simulink model "four_CIFF_EM_sim"  (R2020a)
settings: Solver=VariableStepAuto  StartTime=0.0  StopTime=0.2  MaxStep=1.55424749113179e-06  RelTol=0.0001
values from neighbouring files (symbols this model uses):
  a = [1 -1]    [CIC_Filter.m]    (also in Cascade_CIC_Filter.m; four_CIFF_EM.m = 0.9)
  Amax = 8    [four_CIFF_EM.m]
  Amp1 = 10*5.13e-6    (= 5.13e-05)    [four_CIFF_EM.m]
  finrad = Fin*2*pi    (= 188.495559215)    [four_CIFF_EM.m]
  g1 = 0.4    [four_CIFF_EM.m]
  g2 = 0.2    [four_CIFF_EM.m]
  g3 = 4    [four_CIFF_EM.m]
  g4 = 0.9    [four_CIFF_EM.m]
  GAIN = 50    [four_CIFF_EM.m]
  Kcv = 4e12    (= 4000000000000)    [four_CIFF_EM.m]
  Kvf = 1.323e-4    (= 0.0001323)    [four_CIFF_EM.m]
  n = length(w)    [CIC_Filter.m]    (also in Cascade_CIC_Filter.m; Half_Band_Filter.m = 18; four_CIFF_EM.m = 0.08)
  Ts = 1/Fs    (= 1.953125e-06)    [four_CIFF_EM.m]
  Vref = 1    [four_CIFF_EM.m]
  ws = sqrt(k/m)    [four_CIFF_EM.m]
libraries: SDtoolbox x1
(part 1 of 3)
settings Model: Creator=Chuqby  LastModifiedBy=Chuqby
settings DataIOCC: ReturnWorkspaceOutputs=off

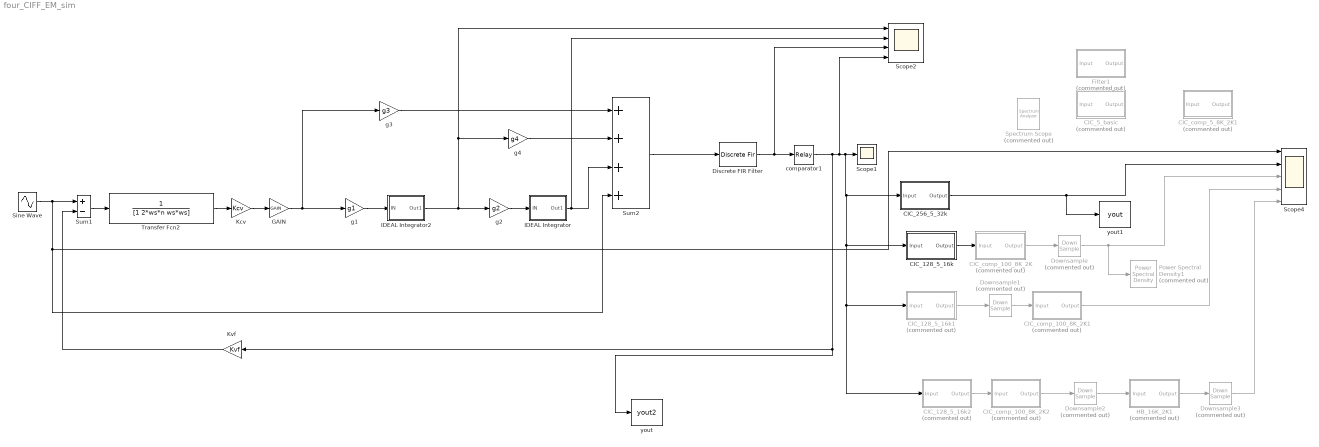
== system four_CIFF_EM_sim ==
  CIC_128_5_16k : Subsystem  Tag=FilterWizardSubSystem
      settings: ErrorFcn=dspFilterRealizedInBasicElemsAlgLoopErrFcnCallback
  CIC_128_5_16k1 : Subsystem  Tag=FilterWizardSubSystem  Commented=on
      settings: ErrorFcn=dspFilterRealizedInBasicElemsAlgLoopErrFcnCallback
  CIC_128_5_16k2 : Subsystem  Tag=FilterWizardSubSystem  Commented=on
      settings: ErrorFcn=dspFilterRealizedInBasicElemsAlgLoopErrFcnCallback
  CIC_256_5_32k : Subsystem  Tag=FilterWizardSubSystem
      settings: ErrorFcn=dspFilterRealizedInBasicElemsAlgLoopErrFcnCallback
  CIC_5_basic : Subsystem  Tag=FilterWizardSubSystem  Commented=on
      settings: ErrorFcn=dspFilterRealizedInBasicElemsAlgLoopErrFcnCallback
  CIC_comp_100_8K_2K : Subsystem  Tag=FilterWizardSubSystem  Commented=on
      settings: ErrorFcn=dspFilterRealizedInBasicElemsAlgLoopErrFcnCallback
  CIC_comp_100_8K_2K1 : Subsystem  Tag=FilterWizardSubSystem  Commented=on
      settings: ErrorFcn=dspFilterRealizedInBasicElemsAlgLoopErrFcnCallback
  CIC_comp_100_8K_2K2 : Subsystem  Tag=FilterWizardSubSystem  Commented=on
      settings: ErrorFcn=dspFilterRealizedInBasicElemsAlgLoopErrFcnCallback
  CIC_comp_5_8K_2K1 : Subsystem  Tag=FilterWizardSubSystem  Commented=on
      settings: ErrorFcn=dspFilterRealizedInBasicElemsAlgLoopErrFcnCallback
  Discrete FIR Filter : DiscreteFir  Coefficients=[1 -a]  SampleTime=Ts
  Downsample{,1..3} (4 alike) : DownSample  Commented=on  RateOptions=Allow multirate processing
  Filter1 : Subsystem  Tag=FilterWizardSubSystem  Commented=on
      settings: ErrorFcn=dspFilterRealizedInBasicElemsAlgLoopErrFcnCallback
  GAIN : Gain  Gain=GAIN
  HB_16K_2K1 : Subsystem  Tag=FilterWizardSubSystem  Commented=on
      settings: ErrorFcn=dspFilterRealizedInBasicElemsAlgLoopErrFcnCallback
  IDEAL Integrator : Subsystem  mask(Integrator){Amax=Amax, Ts=Ts}
      mask prompts: Amax "Saturation"; Ts "Sample Time:"
      mask help:
      | Real discrete integrator with delay.
      | Models op-amp saturation and slew rate.
      mask Help:
      | Parameters:
      | Ts:       Sample time
      | G:         Finite op-amp gain (ideal op-amp G=1)
      | Amax:  Saturation value
      | sr:       slew rate in V/s
      mask Display: dpoly([0 1], [1 -1], 'z-')
  IDEAL Integrator2 : Subsystem  mask(Integrator){Amax=Amax, Ts=Ts}
      mask prompts: Amax "Saturation"; Ts "Sample Time:"
      mask help:
      | Real discrete integrator with delay.
      | Models op-amp saturation and slew rate.
      mask Help:
      | Parameters:
      | Ts:       Sample time
      | G:         Finite op-amp gain (ideal op-amp G=1)
      | Amax:  Saturation value
      | sr:       slew rate in V/s
      mask Display: dpoly([0 1], [1 -1], 'z-')
  Kcv : Gain  Gain=Kcv
  Kvf : Gain  Gain=Kvf
  Power Spectral Density1 : SDtoolbox/Power Spectral Density  Commented=on  SN=1  Fs=8000  fBL=1  fBH=2000  Fin=30  N=65535  Ntransient=Ntransient  VW=off  savename=savemat  Scale_type=logarithmic
  Scope1 : Scope
  Scope2 : Scope  NumInputPorts=4
  Scope4 : Scope  NumInputPorts=5
  Sine Wave : Sin  Amplitude=Amp1  Frequency=finrad  SampleTime=0
  Spectrum Scope : SpectrumAnalyzer  Commented=on
  Sum1 : Sum  Inputs=+-
  Sum2 : Sum  Inputs=++++
  Transfer Fcn2 : TransferFcn  Denominator=[1 2*ws*n ws*ws]
  comparator1 : Relay  OnOutputValue=Vref  OffOutputValue=-Vref  ZeroCross=off
  g1 : Gain  Gain=g1
  g2 : Gain  Gain=g2
  g3 : Gain  Gain=g3
  g4 : Gain  Gain=g4
  yout : ToWorkspace  VariableName=yout2  SampleTime=-1
      settings: Save2DSignal=2-D array (concatenate along first dimension)
  yout1 : ToWorkspace  VariableName=yout  SampleTime=-1
      settings: Save2DSignal=2-D array (concatenate along first dimension)
  wires:
  IDEAL Integrator2/1(Out1) -> Scope2/1, g4/1, g2/1
  g3/1 -> Sum2/1
  g4/1 -> Sum2/2
  Sum1/1 -> Transfer Fcn2/1
  Discrete FIR Filter/1 -> Scope2/3, comparator1/1
  g1/1 -> IDEAL Integrator2/1(IN)
  g2/1 -> IDEAL Integrator/1(IN)
  Sum2/1 -> Discrete FIR Filter/1
  Transfer Fcn2/1 -> Kcv/1
  IDEAL Integrator/1(Out1) -> Sum2/3, Scope2/2
  Sine Wave/1 -> Scope4/1, Sum2/4, Sum1/1
  Kcv/1 -> GAIN/1
  comparator1/1 -> Scope2/4, CIC_256_5_32k/1(Input), CIC_128_5_16k2/1(Input), CIC_128_5_16k1/1(Input), CIC_128_5_16k/1(Input), Scope1/1, yout/1, Kvf/1
  GAIN/1 -> g1/1, g3/1
  Kvf/1 -> Sum1/2
  CIC_256_5_32k/1(Output) -> yout1/1, Scope4/2
  CIC_128_5_16k/1(Output) -> CIC_comp_100_8K_2K/1(Input)
  CIC_comp_100_8K_2K/1(Output) -> Downsample/1
  Downsample/1 -> Power Spectral Density1/1, Scope4/3
  CIC_128_5_16k1/1(Output) -> Downsample1/1
  Downsample1/1 -> CIC_comp_100_8K_2K1/1(Input)
  CIC_comp_100_8K_2K1/1(Output) -> Scope4/4
  CIC_comp_100_8K_2K2/1(Output) -> Downsample2/1
  CIC_128_5_16k2/1(Output) -> CIC_comp_100_8K_2K2/1(Input)
  Downsample2/1 -> HB_16K_2K1/1(Input)
  Downsample3/1 -> Scope4/5
  HB_16K_2K1/1(Output) -> Downsample3/1

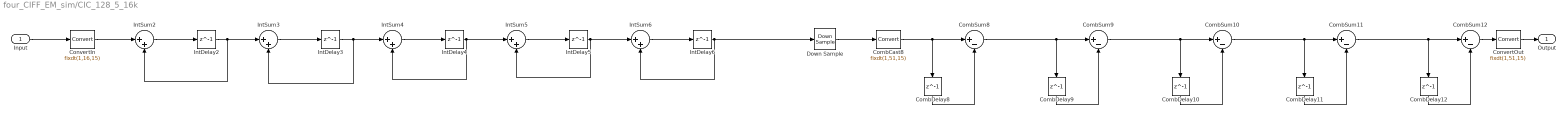
== system four_CIFF_EM_sim/CIC_128_5_16k ==
  Input : Inport
  CombCast8 : DataTypeConversion  OutDataTypeStr=fixdt(1,51,15)
  CombDelay{8..12} (5 alike) : Delay  DelayLength=1  InitialCondition=0
  CombSum{8..12} (5 alike) : Sum  Inputs=|+-  AccumDataTypeStr=fixdt(1,51,15)  OutDataTypeStr=fixdt(1,51,15)
  ConvertIn : DataTypeConversion  OutDataTypeStr=fixdt(1,16,15)  RndMeth=Nearest  SaturateOnIntegerOverflow=on
  ConvertOut : DataTypeConversion  OutDataTypeStr=fixdt(1,51,15)
  Down Sample : DownSample  N=128  RateOptions=Allow multirate processing
  IntDelay{2..6} (5 alike) : Delay  DelayLength=1  InitialCondition=0
  IntSum{2..6} (5 alike) : Sum  Inputs=|++  AccumDataTypeStr=fixdt(1,51,15)  OutDataTypeStr=fixdt(1,51,15)
  Output : Outport
  wires:
  Input/1 -> ConvertIn/1
  ConvertIn/1 -> IntSum2/1
  IntSum2/1 -> IntDelay2/1
  IntDelay2/1 -> IntSum2/2, IntSum3/1
  IntSum3/1 -> IntDelay3/1
  IntDelay3/1 -> IntSum3/2, IntSum4/1
  IntSum4/1 -> IntDelay4/1
  IntDelay4/1 -> IntSum4/2, IntSum5/1
  IntSum5/1 -> IntDelay5/1
  IntDelay5/1 -> IntSum5/2, IntSum6/1
  IntSum6/1 -> IntDelay6/1
  IntDelay6/1 -> IntSum6/2, Down Sample/1
  Down Sample/1 -> CombCast8/1
  CombSum8/1 -> CombSum9/1, CombDelay9/1
  CombDelay8/1 -> CombSum8/2
  CombCast8/1 -> CombSum8/1, CombDelay8/1
  CombSum9/1 -> CombSum10/1, CombDelay10/1
  CombDelay9/1 -> CombSum9/2
  CombSum10/1 -> CombSum11/1, CombDelay11/1
  CombDelay10/1 -> CombSum10/2
  CombSum11/1 -> CombSum12/1, CombDelay12/1
  CombDelay11/1 -> CombSum11/2
  CombSum12/1 -> ConvertOut/1
  CombDelay12/1 -> CombSum12/2
  ConvertOut/1 -> Output/1

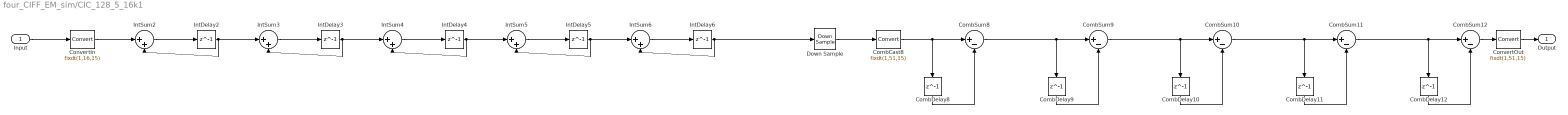
== system four_CIFF_EM_sim/CIC_128_5_16k1 ==
  Input : Inport
  CombCast8 : DataTypeConversion  OutDataTypeStr=fixdt(1,51,15)
  CombDelay{8..12} (5 alike) : Delay  DelayLength=1  InitialCondition=0
  CombSum{8..12} (5 alike) : Sum  Inputs=|+-  AccumDataTypeStr=fixdt(1,51,15)  OutDataTypeStr=fixdt(1,51,15)
  ConvertIn : DataTypeConversion  OutDataTypeStr=fixdt(1,16,15)  RndMeth=Nearest  SaturateOnIntegerOverflow=on
  ConvertOut : DataTypeConversion  OutDataTypeStr=fixdt(1,51,15)
  Down Sample : DownSample  N=128  RateOptions=Allow multirate processing
  IntDelay{2..6} (5 alike) : Delay  DelayLength=1  InitialCondition=0
  IntSum{2..6} (5 alike) : Sum  Inputs=|++  AccumDataTypeStr=fixdt(1,51,15)  OutDataTypeStr=fixdt(1,51,15)
  Output : Outport
  wires:
  ConvertOut/1 -> Output/1
  CombDelay12/1 -> CombSum12/2
  CombSum12/1 -> ConvertOut/1
  CombDelay11/1 -> CombSum11/2
  CombSum11/1 -> CombDelay12/1, CombSum12/1
  CombDelay10/1 -> CombSum10/2
  CombSum10/1 -> CombDelay11/1, CombSum11/1
  CombDelay9/1 -> CombSum9/2
  CombSum9/1 -> CombDelay10/1, CombSum10/1
  CombCast8/1 -> CombDelay8/1, CombSum8/1
  CombDelay8/1 -> CombSum8/2
  CombSum8/1 -> CombDelay9/1, CombSum9/1
  Down Sample/1 -> CombCast8/1
  IntDelay6/1 -> Down Sample/1, IntSum6/2
  IntSum6/1 -> IntDelay6/1
  IntDelay5/1 -> IntSum6/1, IntSum5/2
  IntSum5/1 -> IntDelay5/1
  IntDelay4/1 -> IntSum5/1, IntSum4/2
  IntSum4/1 -> IntDelay4/1
  IntDelay3/1 -> IntSum4/1, IntSum3/2
  IntSum3/1 -> IntDelay3/1
  IntDelay2/1 -> IntSum3/1, IntSum2/2
  IntSum2/1 -> IntDelay2/1
  ConvertIn/1 -> IntSum2/1
  Input/1 -> ConvertIn/1

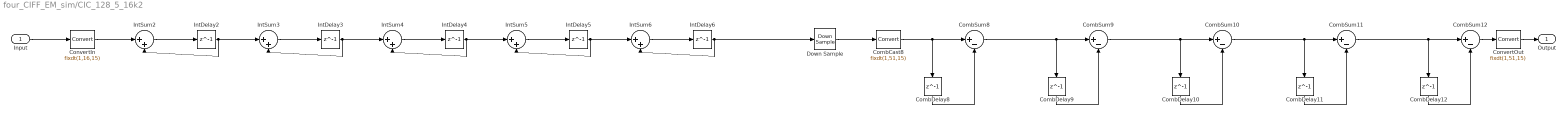
== system four_CIFF_EM_sim/CIC_128_5_16k2 ==
  Input : Inport
  CombCast8 : DataTypeConversion  OutDataTypeStr=fixdt(1,51,15)
  CombDelay{8..12} (5 alike) : Delay  DelayLength=1  InitialCondition=0
  CombSum{8..12} (5 alike) : Sum  Inputs=|+-  AccumDataTypeStr=fixdt(1,51,15)  OutDataTypeStr=fixdt(1,51,15)
  ConvertIn : DataTypeConversion  OutDataTypeStr=fixdt(1,16,15)  RndMeth=Nearest  SaturateOnIntegerOverflow=on
  ConvertOut : DataTypeConversion  OutDataTypeStr=fixdt(1,51,15)
  Down Sample : DownSample  N=128  RateOptions=Allow multirate processing
  IntDelay{2..6} (5 alike) : Delay  DelayLength=1  InitialCondition=0
  IntSum{2..6} (5 alike) : Sum  Inputs=|++  AccumDataTypeStr=fixdt(1,51,15)  OutDataTypeStr=fixdt(1,51,15)
  Output : Outport
  wires:
  Input/1 -> ConvertIn/1
  ConvertIn/1 -> IntSum2/1
  IntSum2/1 -> IntDelay2/1
  IntDelay2/1 -> IntSum2/2, IntSum3/1
  IntSum3/1 -> IntDelay3/1
  IntDelay3/1 -> IntSum3/2, IntSum4/1
  IntSum4/1 -> IntDelay4/1
  IntDelay4/1 -> IntSum4/2, IntSum5/1
  IntSum5/1 -> IntDelay5/1
  IntDelay5/1 -> IntSum5/2, IntSum6/1
  IntSum6/1 -> IntDelay6/1
  IntDelay6/1 -> IntSum6/2, Down Sample/1
  Down Sample/1 -> CombCast8/1
  CombSum8/1 -> CombSum9/1, CombDelay9/1
  CombDelay8/1 -> CombSum8/2
  CombCast8/1 -> CombSum8/1, CombDelay8/1
  CombSum9/1 -> CombSum10/1, CombDelay10/1
  CombDelay9/1 -> CombSum9/2
  CombSum10/1 -> CombSum11/1, CombDelay11/1
  CombDelay10/1 -> CombSum10/2
  CombSum11/1 -> CombSum12/1, CombDelay12/1
  CombDelay11/1 -> CombSum11/2
  CombSum12/1 -> ConvertOut/1
  CombDelay12/1 -> CombSum12/2
  ConvertOut/1 -> Output/1

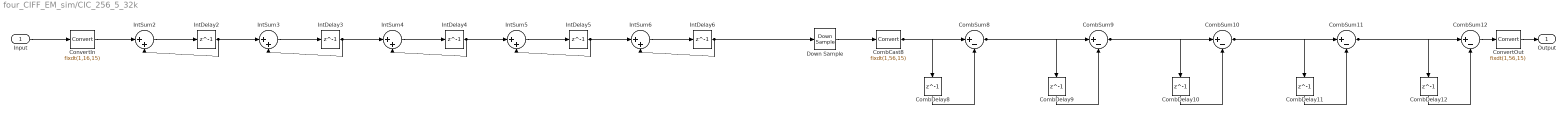
== system four_CIFF_EM_sim/CIC_256_5_32k ==
  Input : Inport
  CombCast8 : DataTypeConversion  OutDataTypeStr=fixdt(1,56,15)
  CombDelay{8..12} (5 alike) : Delay  DelayLength=1  InitialCondition=0
  CombSum{8..12} (5 alike) : Sum  Inputs=|+-  AccumDataTypeStr=fixdt(1,56,15)  OutDataTypeStr=fixdt(1,56,15)
  ConvertIn : DataTypeConversion  OutDataTypeStr=fixdt(1,16,15)  RndMeth=Nearest  SaturateOnIntegerOverflow=on
  ConvertOut : DataTypeConversion  OutDataTypeStr=fixdt(1,56,15)
  Down Sample : DownSample  N=256  RateOptions=Allow multirate processing
  IntDelay{2..6} (5 alike) : Delay  DelayLength=1  InitialCondition=0
  IntSum{2..6} (5 alike) : Sum  Inputs=|++  AccumDataTypeStr=fixdt(1,56,15)  OutDataTypeStr=fixdt(1,56,15)
  Output : Outport
  wires:
  Input/1 -> ConvertIn/1
  ConvertIn/1 -> IntSum2/1
  IntSum2/1 -> IntDelay2/1
  IntDelay2/1 -> IntSum2/2, IntSum3/1
  IntSum3/1 -> IntDelay3/1
  IntDelay3/1 -> IntSum3/2, IntSum4/1
  IntSum4/1 -> IntDelay4/1
  IntDelay4/1 -> IntSum4/2, IntSum5/1
  IntSum5/1 -> IntDelay5/1
  IntDelay5/1 -> IntSum5/2, IntSum6/1
  IntSum6/1 -> IntDelay6/1
  IntDelay6/1 -> IntSum6/2, Down Sample/1
  Down Sample/1 -> CombCast8/1
  CombSum8/1 -> CombSum9/1, CombDelay9/1
  CombDelay8/1 -> CombSum8/2
  CombCast8/1 -> CombSum8/1, CombDelay8/1
  CombSum9/1 -> CombSum10/1, CombDelay10/1
  CombDelay9/1 -> CombSum9/2
  CombSum10/1 -> CombSum11/1, CombDelay11/1
  CombDelay10/1 -> CombSum10/2
  CombSum11/1 -> CombSum12/1, CombDelay12/1
  CombDelay11/1 -> CombSum11/2
  CombSum12/1 -> ConvertOut/1
  CombDelay12/1 -> CombSum12/2
  ConvertOut/1 -> Output/1

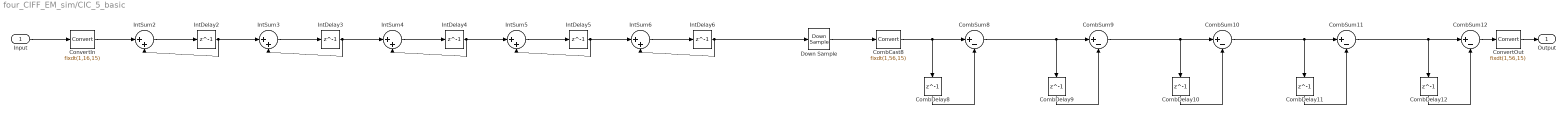
== system four_CIFF_EM_sim/CIC_5_basic ==
  Input : Inport
  CombCast8 : DataTypeConversion  OutDataTypeStr=fixdt(1,56,15)
  CombDelay{8..12} (5 alike) : Delay  DelayLength=1  InitialCondition=0
  CombSum{8..12} (5 alike) : Sum  Inputs=|+-  AccumDataTypeStr=fixdt(1,56,15)  OutDataTypeStr=fixdt(1,56,15)
  ConvertIn : DataTypeConversion  OutDataTypeStr=fixdt(1,16,15)  RndMeth=Nearest  SaturateOnIntegerOverflow=on
  ConvertOut : DataTypeConversion  OutDataTypeStr=fixdt(1,56,15)
  Down Sample : DownSample  N=256  RateOptions=Allow multirate processing
  IntDelay{2..6} (5 alike) : Delay  DelayLength=1  InitialCondition=0
  IntSum{2..6} (5 alike) : Sum  Inputs=|++  AccumDataTypeStr=fixdt(1,56,15)  OutDataTypeStr=fixdt(1,56,15)
  Output : Outport
  wires:
  Input/1 -> ConvertIn/1
  ConvertIn/1 -> IntSum2/1
  IntSum2/1 -> IntDelay2/1
  IntDelay2/1 -> IntSum2/2, IntSum3/1
  IntSum3/1 -> IntDelay3/1
  IntDelay3/1 -> IntSum3/2, IntSum4/1
  IntSum4/1 -> IntDelay4/1
  IntDelay4/1 -> IntSum4/2, IntSum5/1
  IntSum5/1 -> IntDelay5/1
  IntDelay5/1 -> IntSum5/2, IntSum6/1
  IntSum6/1 -> IntDelay6/1
  IntDelay6/1 -> IntSum6/2, Down Sample/1
  Down Sample/1 -> CombCast8/1
  CombSum8/1 -> CombSum9/1, CombDelay9/1
  CombDelay8/1 -> CombSum8/2
  CombCast8/1 -> CombSum8/1, CombDelay8/1
  CombSum9/1 -> CombSum10/1, CombDelay10/1
  CombDelay9/1 -> CombSum9/2
  CombSum10/1 -> CombSum11/1, CombDelay11/1
  CombDelay10/1 -> CombSum10/2
  CombSum11/1 -> CombSum12/1, CombDelay12/1
  CombDelay11/1 -> CombSum11/2
  CombSum12/1 -> ConvertOut/1
  CombDelay12/1 -> CombSum12/2
  ConvertOut/1 -> Output/1

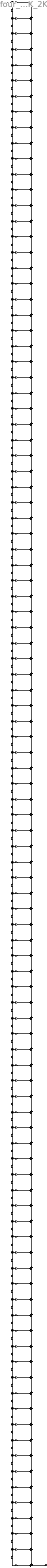
== system four_CIFF_EM_sim/CIC_comp_100_8K_2K ==
  Input : Inport
  BodyDelay{2..101} (100 alike) : Delay  DelayLength=1  InitialCondition=0
  BodyLSum{2..101} (100 alike) : Sum  Inputs=++|  RndMeth=Nearest  SaturateOnIntegerOverflow=on  OutDataTypeStr=Inherit: Same as first input
  b(1) : Gain  Gain=-1.79724995551988194e-05  ParamDataTypeStr=double  RndMeth=Nearest  SaturateOnIntegerOverflow=on  OutDataTypeStr=Inherit: Same as input
  b(10) : Gain  Gain=-0.00135713674496342439  ParamDataTypeStr=double  RndMeth=Nearest  SaturateOnIntegerOverflow=on  OutDataTypeStr=Inherit: Same as input
  b(100) : Gain  Gain=0.000217864908938036016  ParamDataTypeStr=double  RndMeth=Nearest  SaturateOnIntegerOverflow=on  OutDataTypeStr=Inherit: Same as input
  b(101) : Gain  Gain=-1.79724995551988194e-05  ParamDataTypeStr=double  RndMeth=Nearest  SaturateOnIntegerOverflow=on  OutDataTypeStr=Inherit: Same as input
  b(11) : Gain  Gain=-0.000789454956120377188  ParamDataTypeStr=double  RndMeth=Nearest  SaturateOnIntegerOverflow=on  OutDataTypeStr=Inherit: Same as input
  b(12) : Gain  Gain=0.00186982608138826288  ParamDataTypeStr=double  RndMeth=Nearest  SaturateOnIntegerOverflow=on  OutDataTypeStr=Inherit: Same as input
  b(13) : Gain  Gain=0.000759222469644703596  ParamDataTypeStr=double  RndMeth=Nearest  SaturateOnIntegerOverflow=on  OutDataTypeStr=Inherit: Same as input
  b(14) : Gain  Gain=-0.00253720373381599628  ParamDataTypeStr=double  RndMeth=Nearest  SaturateOnIntegerOverflow=on  OutDataTypeStr=Inherit: Same as input
  b(15) : Gain  Gain=-0.000590518576863596658  ParamDataTypeStr=double  RndMeth=Nearest  SaturateOnIntegerOverflow=on  OutDataTypeStr=Inherit: Same as input
  b(16) : Gain  Gain=0.00335428953613474239  ParamDataTypeStr=double  RndMeth=Nearest  SaturateOnIntegerOverflow=on  OutDataTypeStr=Inherit: Same as input
  b(17) : Gain  Gain=0.000204368164461546018  ParamDataTypeStr=double  RndMeth=Nearest  SaturateOnIntegerOverflow=on  OutDataTypeStr=Inherit: Same as input
  b(18) : Gain  Gain=-0.00429941158795879574  ParamDataTypeStr=double  RndMeth=Nearest  SaturateOnIntegerOverflow=on  OutDataTypeStr=Inherit: Same as input
  b(19) : Gain  Gain=0.000485636343031858625  ParamDataTypeStr=double  RndMeth=Nearest  SaturateOnIntegerOverflow=on  OutDataTypeStr=Inherit: Same as input
  b(2) : Gain  Gain=0.000217864908938036016  ParamDataTypeStr=double  RndMeth=Nearest  SaturateOnIntegerOverflow=on  OutDataTypeStr=Inherit: Same as input
  b(20) : Gain  Gain=0.00532504087437809821  ParamDataTypeStr=double  RndMeth=Nearest  SaturateOnIntegerOverflow=on  OutDataTypeStr=Inherit: Same as input
  b(21) : Gain  Gain=-0.00156923303295267136  ParamDataTypeStr=double  RndMeth=Nearest  SaturateOnIntegerOverflow=on  OutDataTypeStr=Inherit: Same as input
  b(22) : Gain  Gain=-0.00635123193963801121  ParamDataTypeStr=double  RndMeth=Nearest  SaturateOnIntegerOverflow=on  OutDataTypeStr=Inherit: Same as input
  b(23) : Gain  Gain=0.0031328343655890635  ParamDataTypeStr=double  RndMeth=Nearest  SaturateOnIntegerOverflow=on  OutDataTypeStr=Inherit: Same as input
  b(24) : Gain  Gain=0.00726140785091971847  ParamDataTypeStr=double  RndMeth=Nearest  SaturateOnIntegerOverflow=on  OutDataTypeStr=Inherit: Same as input
  b(25) : Gain  Gain=-0.00525092869031457826  ParamDataTypeStr=double  RndMeth=Nearest  SaturateOnIntegerOverflow=on  OutDataTypeStr=Inherit: Same as input
  b(26) : Gain  Gain=-0.00790051120858381584  ParamDataTypeStr=double  RndMeth=Nearest  SaturateOnIntegerOverflow=on  OutDataTypeStr=Inherit: Same as input
  b(27) : Gain  Gain=0.00797633219974696467  ParamDataTypeStr=double  RndMeth=Nearest  SaturateOnIntegerOverflow=on  OutDataTypeStr=Inherit: Same as input
  b(28) : Gain  Gain=0.0080749829489765515  ParamDataTypeStr=double  RndMeth=Nearest  SaturateOnIntegerOverflow=on  OutDataTypeStr=Inherit: Same as input
  b(29) : Gain  Gain=-0.0113308252747029853  ParamDataTypeStr=double  RndMeth=Nearest  SaturateOnIntegerOverflow=on  OutDataTypeStr=Inherit: Same as input
  b(3) : Gain  Gain=0.00101657656543529401  ParamDataTypeStr=double  RndMeth=Nearest  SaturateOnIntegerOverflow=on  OutDataTypeStr=Inherit: Same as input
  b(30) : Gain  Gain=-0.00755365464854574481  ParamDataTypeStr=double  RndMeth=Nearest  SaturateOnIntegerOverflow=on  OutDataTypeStr=Inherit: Same as input
  b(31) : Gain  Gain=0.0152980505107621519  ParamDataTypeStr=double  RndMeth=Nearest  SaturateOnIntegerOverflow=on  OutDataTypeStr=Inherit: Same as input
  b(32) : Gain  Gain=0.00606784749975600255  ParamDataTypeStr=double  RndMeth=Nearest  SaturateOnIntegerOverflow=on  OutDataTypeStr=Inherit: Same as input
  b(33) : Gain  Gain=-0.0198205266353495731  ParamDataTypeStr=double  RndMeth=Nearest  SaturateOnIntegerOverflow=on  OutDataTypeStr=Inherit: Same as input
  b(34) : Gain  Gain=-0.00330711838882566866  ParamDataTypeStr=double  RndMeth=Nearest  SaturateOnIntegerOverflow=on  OutDataTypeStr=Inherit: Same as input
  b(35) : Gain  Gain=0.0248026071466539537  ParamDataTypeStr=double  RndMeth=Nearest  SaturateOnIntegerOverflow=on  OutDataTypeStr=Inherit: Same as input
  b(36) : Gain  Gain=-0.00109692464626924969  ParamDataTypeStr=double  RndMeth=Nearest  SaturateOnIntegerOverflow=on  OutDataTypeStr=Inherit: Same as input
  b(37) : Gain  Gain=-0.030122109433535018  ParamDataTypeStr=double  RndMeth=Nearest  SaturateOnIntegerOverflow=on  OutDataTypeStr=Inherit: Same as input
  b(38) : Gain  Gain=0.00761482085988017879  ParamDataTypeStr=double  RndMeth=Nearest  SaturateOnIntegerOverflow=on  OutDataTypeStr=Inherit: Same as input
  b(39) : Gain  Gain=0.0356568893392657099  ParamDataTypeStr=double  RndMeth=Nearest  SaturateOnIntegerOverflow=on  OutDataTypeStr=Inherit: Same as input
  b(4) : Gain  Gain=0.00165871902897375147  ParamDataTypeStr=double  RndMeth=Nearest  SaturateOnIntegerOverflow=on  OutDataTypeStr=Inherit: Same as input
  b(40) : Gain  Gain=-0.0169277110938957955  ParamDataTypeStr=double  RndMeth=Nearest  SaturateOnIntegerOverflow=on  OutDataTypeStr=Inherit: Same as input
  b(41) : Gain  Gain=-0.0413436765687130656  ParamDataTypeStr=double  RndMeth=Nearest  SaturateOnIntegerOverflow=on  OutDataTypeStr=Inherit: Same as input
  b(42) : Gain  Gain=0.0301937311298770342  ParamDataTypeStr=double  RndMeth=Nearest  SaturateOnIntegerOverflow=on  OutDataTypeStr=Inherit: Same as input
  b(43) : Gain  Gain=0.0473262085121037429  ParamDataTypeStr=double  RndMeth=Nearest  SaturateOnIntegerOverflow=on  OutDataTypeStr=Inherit: Same as input
  b(44) : Gain  Gain=-0.0497599250874532356  ParamDataTypeStr=double  RndMeth=Nearest  SaturateOnIntegerOverflow=on  OutDataTypeStr=Inherit: Same as input
  b(45) : Gain  Gain=-0.0544238724208939428  ParamDataTypeStr=double  RndMeth=Nearest  SaturateOnIntegerOverflow=on  OutDataTypeStr=Inherit: Same as input
  b(46) : Gain  Gain=0.0814225100528190998  ParamDataTypeStr=double  RndMeth=Nearest  SaturateOnIntegerOverflow=on  OutDataTypeStr=Inherit: Same as input
  b(47) : Gain  Gain=0.0661921425209298919  ParamDataTypeStr=double  RndMeth=Nearest  SaturateOnIntegerOverflow=on  OutDataTypeStr=Inherit: Same as input
  b(48) : Gain  Gain=-0.144076313546327328  ParamDataTypeStr=double  RndMeth=Nearest  SaturateOnIntegerOverflow=on  OutDataTypeStr=Inherit: Same as input
  b(49) : Gain  Gain=-0.10417685895098662  ParamDataTypeStr=double  RndMeth=Nearest  SaturateOnIntegerOverflow=on  OutDataTypeStr=Inherit: Same as input
  b(5) : Gain  Gain=0.000798403729563677638  ParamDataTypeStr=double  RndMeth=Nearest  SaturateOnIntegerOverflow=on  OutDataTypeStr=Inherit: Same as input
  b(50) : Gain  Gain=0.343411075679583622  ParamDataTypeStr=double  RndMeth=Nearest  SaturateOnIntegerOverflow=on  OutDataTypeStr=Inherit: Same as input
  b(51) : Gain  Gain=0.634384304400381627  ParamDataTypeStr=double  RndMeth=Nearest  SaturateOnIntegerOverflow=on  OutDataTypeStr=Inherit: Same as input
  b(52) : Gain  Gain=0.343411075679583622  ParamDataTypeStr=double  RndMeth=Nearest  SaturateOnIntegerOverflow=on  OutDataTypeStr=Inherit: Same as input
  b(53) : Gain  Gain=-0.10417685895098662  ParamDataTypeStr=double  RndMeth=Nearest  SaturateOnIntegerOverflow=on  OutDataTypeStr=Inherit: Same as input
  b(54) : Gain  Gain=-0.144076313546327328  ParamDataTypeStr=double  RndMeth=Nearest  SaturateOnIntegerOverflow=on  OutDataTypeStr=Inherit: Same as input
  b(55) : Gain  Gain=0.0661921425209298919  ParamDataTypeStr=double  RndMeth=Nearest  SaturateOnIntegerOverflow=on  OutDataTypeStr=Inherit: Same as input
  b(56) : Gain  Gain=0.0814225100528190998  ParamDataTypeStr=double  RndMeth=Nearest  SaturateOnIntegerOverflow=on  OutDataTypeStr=Inherit: Same as input
  b(57) : Gain  Gain=-0.0544238724208939428  ParamDataTypeStr=double  RndMeth=Nearest  SaturateOnIntegerOverflow=on  OutDataTypeStr=Inherit: Same as input
  b(58) : Gain  Gain=-0.0497599250874532356  ParamDataTypeStr=double  RndMeth=Nearest  SaturateOnIntegerOverflow=on  OutDataTypeStr=Inherit: Same as input
  b(59) : Gain  Gain=0.0473262085121037429  ParamDataTypeStr=double  RndMeth=Nearest  SaturateOnIntegerOverflow=on  OutDataTypeStr=Inherit: Same as input
  b(6) : Gain  Gain=-0.000865780464857189439  ParamDataTypeStr=double  RndMeth=Nearest  SaturateOnIntegerOverflow=on  OutDataTypeStr=Inherit: Same as input
  b(60) : Gain  Gain=0.0301937311298770342  ParamDataTypeStr=double  RndMeth=Nearest  SaturateOnIntegerOverflow=on  OutDataTypeStr=Inherit: Same as input
  b(61) : Gain  Gain=-0.0413436765687130656  ParamDataTypeStr=double  RndMeth=Nearest  SaturateOnIntegerOverflow=on  OutDataTypeStr=Inherit: Same as input
  b(62) : Gain  Gain=-0.0169277110938957955  ParamDataTypeStr=double  RndMeth=Nearest  SaturateOnIntegerOverflow=on  OutDataTypeStr=Inherit: Same as input
  b(63) : Gain  Gain=0.0356568893392657099  ParamDataTypeStr=double  RndMeth=Nearest  SaturateOnIntegerOverflow=on  OutDataTypeStr=Inherit: Same as input
  b(64) : Gain  Gain=0.00761482085988017879  ParamDataTypeStr=double  RndMeth=Nearest  SaturateOnIntegerOverflow=on  OutDataTypeStr=Inherit: Same as input
  b(65) : Gain  Gain=-0.030122109433535018  ParamDataTypeStr=double  RndMeth=Nearest  SaturateOnIntegerOverflow=on  OutDataTypeStr=Inherit: Same as input
  b(66) : Gain  Gain=-0.00109692464626924969  ParamDataTypeStr=double  RndMeth=Nearest  SaturateOnIntegerOverflow=on  OutDataTypeStr=Inherit: Same as input
  b(67) : Gain  Gain=0.0248026071466539537  ParamDataTypeStr=double  RndMeth=Nearest  SaturateOnIntegerOverflow=on  OutDataTypeStr=Inherit: Same as input
  b(68) : Gain  Gain=-0.00330711838882566866  ParamDataTypeStr=double  RndMeth=Nearest  SaturateOnIntegerOverflow=on  OutDataTypeStr=Inherit: Same as input
  b(69) : Gain  Gain=-0.0198205266353495731  ParamDataTypeStr=double  RndMeth=Nearest  SaturateOnIntegerOverflow=on  OutDataTypeStr=Inherit: Same as input
  b(7) : Gain  Gain=-0.000721174365704172122  ParamDataTypeStr=double  RndMeth=Nearest  SaturateOnIntegerOverflow=on  OutDataTypeStr=Inherit: Same as input
  b(70) : Gain  Gain=0.00606784749975600255  ParamDataTypeStr=double  RndMeth=Nearest  SaturateOnIntegerOverflow=on  OutDataTypeStr=Inherit: Same as input
  b(71) : Gain  Gain=0.0152980505107621519  ParamDataTypeStr=double  RndMeth=Nearest  SaturateOnIntegerOverflow=on  OutDataTypeStr=Inherit: Same as input
  b(72) : Gain  Gain=-0.00755365464854574481  ParamDataTypeStr=double  RndMeth=Nearest  SaturateOnIntegerOverflow=on  OutDataTypeStr=Inherit: Same as input
  b(73) : Gain  Gain=-0.0113308252747029853  ParamDataTypeStr=double  RndMeth=Nearest  SaturateOnIntegerOverflow=on  OutDataTypeStr=Inherit: Same as input
  b(74) : Gain  Gain=0.0080749829489765515  ParamDataTypeStr=double  RndMeth=Nearest  SaturateOnIntegerOverflow=on  OutDataTypeStr=Inherit: Same as input
  b(75) : Gain  Gain=0.00797633219974696467  ParamDataTypeStr=double  RndMeth=Nearest  SaturateOnIntegerOverflow=on  OutDataTypeStr=Inherit: Same as input
  b(76) : Gain  Gain=-0.00790051120858381584  ParamDataTypeStr=double  RndMeth=Nearest  SaturateOnIntegerOverflow=on  OutDataTypeStr=Inherit: Same as input
  b(77) : Gain  Gain=-0.00525092869031457826  ParamDataTypeStr=double  RndMeth=Nearest  SaturateOnIntegerOverflow=on  OutDataTypeStr=Inherit: Same as input
  b(78) : Gain  Gain=0.00726140785091971847  ParamDataTypeStr=double  RndMeth=Nearest  SaturateOnIntegerOverflow=on  OutDataTypeStr=Inherit: Same as input
  b(79) : Gain  Gain=0.0031328343655890635  ParamDataTypeStr=double  RndMeth=Nearest  SaturateOnIntegerOverflow=on  OutDataTypeStr=Inherit: Same as input
  b(8) : Gain  Gain=0.00100240642691473984  ParamDataTypeStr=double  RndMeth=Nearest  SaturateOnIntegerOverflow=on  OutDataTypeStr=Inherit: Same as input
  b(80) : Gain  Gain=-0.00635123193963801121  ParamDataTypeStr=double  RndMeth=Nearest  SaturateOnIntegerOverflow=on  OutDataTypeStr=Inherit: Same as input
  b(81) : Gain  Gain=-0.00156923303295267136  ParamDataTypeStr=double  RndMeth=Nearest  SaturateOnIntegerOverflow=on  OutDataTypeStr=Inherit: Same as input
  b(82) : Gain  Gain=0.00532504087437809821  ParamDataTypeStr=double  RndMeth=Nearest  SaturateOnIntegerOverflow=on  OutDataTypeStr=Inherit: Same as input
  b(83) : Gain  Gain=0.000485636343031858625  ParamDataTypeStr=double  RndMeth=Nearest  SaturateOnIntegerOverflow=on  OutDataTypeStr=Inherit: Same as input
  b(84) : Gain  Gain=-0.00429941158795879574  ParamDataTypeStr=double  RndMeth=Nearest  SaturateOnIntegerOverflow=on  OutDataTypeStr=Inherit: Same as input
  b(85) : Gain  Gain=0.000204368164461546018  ParamDataTypeStr=double  RndMeth=Nearest  SaturateOnIntegerOverflow=on  OutDataTypeStr=Inherit: Same as input
  b(86) : Gain  Gain=0.00335428953613474239  ParamDataTypeStr=double  RndMeth=Nearest  SaturateOnIntegerOverflow=on  OutDataTypeStr=Inherit: Same as input
  b(87) : Gain  Gain=-0.000590518576863596658  ParamDataTypeStr=double  RndMeth=Nearest  SaturateOnIntegerOverflow=on  OutDataTypeStr=Inherit: Same as input
  b(88) : Gain  Gain=-0.00253720373381599628  ParamDataTypeStr=double  RndMeth=Nearest  SaturateOnIntegerOverflow=on  OutDataTypeStr=Inherit: Same as input
  b(89) : Gain  Gain=0.000759222469644703596  ParamDataTypeStr=double  RndMeth=Nearest  SaturateOnIntegerOverflow=on  OutDataTypeStr=Inherit: Same as input
  b(9) : Gain  Gain=0.000752327125717876439  ParamDataTypeStr=double  RndMeth=Nearest  SaturateOnIntegerOverflow=on  OutDataTypeStr=Inherit: Same as input
  b(90) : Gain  Gain=0.00186982608138826288  ParamDataTypeStr=double  RndMeth=Nearest  SaturateOnIntegerOverflow=on  OutDataTypeStr=Inherit: Same as input
  b(91) : Gain  Gain=-0.000789454956120377188  ParamDataTypeStr=double  RndMeth=Nearest  SaturateOnIntegerOverflow=on  OutDataTypeStr=Inherit: Same as input
  b(92) : Gain  Gain=-0.00135713674496342439  ParamDataTypeStr=double  RndMeth=Nearest  SaturateOnIntegerOverflow=on  OutDataTypeStr=Inherit: Same as input
  b(93) : Gain  Gain=0.000752327125717876439  ParamDataTypeStr=double  RndMeth=Nearest  SaturateOnIntegerOverflow=on  OutDataTypeStr=Inherit: Same as input
  b(94) : Gain  Gain=0.00100240642691473984  ParamDataTypeStr=double  RndMeth=Nearest  SaturateOnIntegerOverflow=on  OutDataTypeStr=Inherit: Same as input
  b(95) : Gain  Gain=-0.000721174365704172122  ParamDataTypeStr=double  RndMeth=Nearest  SaturateOnIntegerOverflow=on  OutDataTypeStr=Inherit: Same as input
  b(96) : Gain  Gain=-0.000865780464857189439  ParamDataTypeStr=double  RndMeth=Nearest  SaturateOnIntegerOverflow=on  OutDataTypeStr=Inherit: Same as input
  b(97) : Gain  Gain=0.000798403729563677638  ParamDataTypeStr=double  RndMeth=Nearest  SaturateOnIntegerOverflow=on  OutDataTypeStr=Inherit: Same as input
  b(98) : Gain  Gain=0.00165871902897375147  ParamDataTypeStr=double  RndMeth=Nearest  SaturateOnIntegerOverflow=on  OutDataTypeStr=Inherit: Same as input
  b(99) : Gain  Gain=0.00101657656543529401  ParamDataTypeStr=double  RndMeth=Nearest  SaturateOnIntegerOverflow=on  OutDataTypeStr=Inherit: Same as input
  Output : Outport
  wires:
  Input/1 -> b(1)/1, BodyDelay2/1
  b(1)/1 -> BodyLSum2/2
  BodyDelay2/1 -> b(2)/1, BodyDelay3/1
  b(2)/1 -> BodyLSum2/1
  BodyLSum2/1 -> BodyLSum3/2
  BodyDelay3/1 -> b(3)/1, BodyDelay4/1
  b(3)/1 -> BodyLSum3/1
  BodyLSum3/1 -> BodyLSum4/2
  BodyDelay4/1 -> b(4)/1, BodyDelay5/1
  b(4)/1 -> BodyLSum4/1
  BodyLSum4/1 -> BodyLSum5/2
  BodyDelay5/1 -> b(5)/1, BodyDelay6/1
  b(5)/1 -> BodyLSum5/1
  BodyLSum5/1 -> BodyLSum6/2
  BodyDelay6/1 -> b(6)/1, BodyDelay7/1
  b(6)/1 -> BodyLSum6/1
  BodyLSum6/1 -> BodyLSum7/2
  BodyDelay7/1 -> b(7)/1, BodyDelay8/1
  b(7)/1 -> BodyLSum7/1
  BodyLSum7/1 -> BodyLSum8/2
  BodyDelay8/1 -> b(8)/1, BodyDelay9/1
  b(8)/1 -> BodyLSum8/1
  BodyLSum8/1 -> BodyLSum9/2
  BodyDelay9/1 -> b(9)/1, BodyDelay10/1
  b(9)/1 -> BodyLSum9/1
  BodyLSum9/1 -> BodyLSum10/2
  BodyDelay10/1 -> b(10)/1, BodyDelay11/1
  b(10)/1 -> BodyLSum10/1
  BodyLSum10/1 -> BodyLSum11/2
  BodyDelay11/1 -> b(11)/1, BodyDelay12/1
  b(11)/1 -> BodyLSum11/1
  BodyLSum11/1 -> BodyLSum12/2
  BodyDelay12/1 -> b(12)/1, BodyDelay13/1
  b(12)/1 -> BodyLSum12/1
  BodyLSum12/1 -> BodyLSum13/2
  BodyDelay13/1 -> b(13)/1, BodyDelay14/1
  b(13)/1 -> BodyLSum13/1
  BodyLSum13/1 -> BodyLSum14/2
  BodyDelay14/1 -> b(14)/1, BodyDelay15/1
  b(14)/1 -> BodyLSum14/1
  BodyLSum14/1 -> BodyLSum15/2
  BodyDelay15/1 -> b(15)/1, BodyDelay16/1
  b(15)/1 -> BodyLSum15/1
  BodyLSum15/1 -> BodyLSum16/2
  BodyDelay16/1 -> b(16)/1, BodyDelay17/1
  b(16)/1 -> BodyLSum16/1
  BodyLSum16/1 -> BodyLSum17/2
  BodyDelay17/1 -> b(17)/1, BodyDelay18/1
  b(17)/1 -> BodyLSum17/1
  BodyLSum17/1 -> BodyLSum18/2
  BodyDelay18/1 -> b(18)/1, BodyDelay19/1
  b(18)/1 -> BodyLSum18/1
  BodyLSum18/1 -> BodyLSum19/2
  BodyDelay19/1 -> b(19)/1, BodyDelay20/1
  b(19)/1 -> BodyLSum19/1
  BodyLSum19/1 -> BodyLSum20/2
  BodyDelay20/1 -> b(20)/1, BodyDelay21/1
  b(20)/1 -> BodyLSum20/1
  BodyLSum20/1 -> BodyLSum21/2
  BodyDelay21/1 -> b(21)/1, BodyDelay22/1
  b(21)/1 -> BodyLSum21/1
  BodyLSum21/1 -> BodyLSum22/2
  BodyDelay22/1 -> b(22)/1, BodyDelay23/1
  b(22)/1 -> BodyLSum22/1
  BodyLSum22/1 -> BodyLSum23/2
  BodyDelay23/1 -> b(23)/1, BodyDelay24/1
  b(23)/1 -> BodyLSum23/1
  BodyLSum23/1 -> BodyLSum24/2
  BodyDelay24/1 -> b(24)/1, BodyDelay25/1
  b(24)/1 -> BodyLSum24/1
  BodyLSum24/1 -> BodyLSum25/2
  BodyDelay25/1 -> b(25)/1, BodyDelay26/1
  b(25)/1 -> BodyLSum25/1
  BodyLSum25/1 -> BodyLSum26/2
  BodyDelay26/1 -> b(26)/1, BodyDelay27/1
  b(26)/1 -> BodyLSum26/1
  BodyLSum26/1 -> BodyLSum27/2
  BodyDelay27/1 -> b(27)/1, BodyDelay28/1
  b(27)/1 -> BodyLSum27/1
  BodyLSum27/1 -> BodyLSum28/2
  BodyDelay28/1 -> b(28)/1, BodyDelay29/1
  b(28)/1 -> BodyLSum28/1
  BodyLSum28/1 -> BodyLSum29/2
  BodyDelay29/1 -> b(29)/1, BodyDelay30/1
  b(29)/1 -> BodyLSum29/1
  BodyLSum29/1 -> BodyLSum30/2
  BodyDelay30/1 -> b(30)/1, BodyDelay31/1
  b(30)/1 -> BodyLSum30/1
  BodyLSum30/1 -> BodyLSum31/2
  BodyDelay31/1 -> b(31)/1, BodyDelay32/1
  b(31)/1 -> BodyLSum31/1
  BodyLSum31/1 -> BodyLSum32/2
  BodyDelay32/1 -> b(32)/1, BodyDelay33/1
  b(32)/1 -> BodyLSum32/1
  BodyLSum32/1 -> BodyLSum33/2
  BodyDelay33/1 -> b(33)/1, BodyDelay34/1
  b(33)/1 -> BodyLSum33/1
  BodyLSum33/1 -> BodyLSum34/2
  BodyDelay34/1 -> b(34)/1, BodyDelay35/1
  b(34)/1 -> BodyLSum34/1
  BodyLSum34/1 -> BodyLSum35/2
  BodyDelay35/1 -> b(35)/1, BodyDelay36/1
  b(35)/1 -> BodyLSum35/1
  BodyLSum35/1 -> BodyLSum36/2
  BodyDelay36/1 -> b(36)/1, BodyDelay37/1
  b(36)/1 -> BodyLSum36/1
  BodyLSum36/1 -> BodyLSum37/2
  BodyDelay37/1 -> b(37)/1, BodyDelay38/1
  b(37)/1 -> BodyLSum37/1
  BodyLSum37/1 -> BodyLSum38/2
  BodyDelay38/1 -> b(38)/1, BodyDelay39/1
  b(38)/1 -> BodyLSum38/1
  BodyLSum38/1 -> BodyLSum39/2
  BodyDelay39/1 -> b(39)/1, BodyDelay40/1
  b(39)/1 -> BodyLSum39/1
  BodyLSum39/1 -> BodyLSum40/2
  BodyDelay40/1 -> b(40)/1, BodyDelay41/1
  b(40)/1 -> BodyLSum40/1
  BodyLSum40/1 -> BodyLSum41/2
  BodyDelay41/1 -> b(41)/1, BodyDelay42/1
  b(41)/1 -> BodyLSum41/1
  BodyLSum41/1 -> BodyLSum42/2
  BodyDelay42/1 -> b(42)/1, BodyDelay43/1
  b(42)/1 -> BodyLSum42/1
  BodyLSum42/1 -> BodyLSum43/2
  BodyDelay43/1 -> b(43)/1, BodyDelay44/1
  b(43)/1 -> BodyLSum43/1
  BodyLSum43/1 -> BodyLSum44/2
  BodyDelay44/1 -> b(44)/1, BodyDelay45/1
  b(44)/1 -> BodyLSum44/1
  BodyLSum44/1 -> BodyLSum45/2
  BodyDelay45/1 -> b(45)/1, BodyDelay46/1
  b(45)/1 -> BodyLSum45/1
  BodyLSum45/1 -> BodyLSum46/2
  BodyDelay46/1 -> b(46)/1, BodyDelay47/1
  b(46)/1 -> BodyLSum46/1
  BodyLSum46/1 -> BodyLSum47/2
  BodyDelay47/1 -> b(47)/1, BodyDelay48/1
  b(47)/1 -> BodyLSum47/1
  BodyLSum47/1 -> BodyLSum48/2
  BodyDelay48/1 -> b(48)/1, BodyDelay49/1
  b(48)/1 -> BodyLSum48/1
  BodyLSum48/1 -> BodyLSum49/2
  BodyDelay49/1 -> b(49)/1, BodyDelay50/1
  b(49)/1 -> BodyLSum49/1
  BodyLSum49/1 -> BodyLSum50/2
  BodyDelay50/1 -> b(50)/1, BodyDelay51/1
  b(50)/1 -> BodyLSum50/1
  BodyLSum50/1 -> BodyLSum51/2
  BodyDelay51/1 -> b(51)/1, BodyDelay52/1
  b(51)/1 -> BodyLSum51/1
  BodyLSum51/1 -> BodyLSum52/2
  BodyDelay52/1 -> b(52)/1, BodyDelay53/1
  b(52)/1 -> BodyLSum52/1
  BodyLSum52/1 -> BodyLSum53/2
  BodyDelay53/1 -> b(53)/1, BodyDelay54/1
  b(53)/1 -> BodyLSum53/1
  BodyLSum53/1 -> BodyLSum54/2
  BodyDelay54/1 -> b(54)/1, BodyDelay55/1
  b(54)/1 -> BodyLSum54/1
  BodyLSum54/1 -> BodyLSum55/2
  BodyDelay55/1 -> b(55)/1, BodyDelay56/1
  b(55)/1 -> BodyLSum55/1
  BodyLSum55/1 -> BodyLSum56/2
  BodyDelay56/1 -> b(56)/1, BodyDelay57/1
  b(56)/1 -> BodyLSum56/1
  BodyLSum56/1 -> BodyLSum57/2
  BodyDelay57/1 -> b(57)/1, BodyDelay58/1
  b(57)/1 -> BodyLSum57/1
  BodyLSum57/1 -> BodyLSum58/2
  BodyDelay58/1 -> b(58)/1, BodyDelay59/1
  b(58)/1 -> BodyLSum58/1
  BodyLSum58/1 -> BodyLSum59/2
  BodyDelay59/1 -> b(59)/1, BodyDelay60/1
  b(59)/1 -> BodyLSum59/1
  BodyLSum59/1 -> BodyLSum60/2
  BodyDelay60/1 -> b(60)/1, BodyDelay61/1
  b(60)/1 -> BodyLSum60/1
  BodyLSum60/1 -> BodyLSum61/2
  BodyDelay61/1 -> b(61)/1, BodyDelay62/1
  b(61)/1 -> BodyLSum61/1
  BodyLSum61/1 -> BodyLSum62/2
  BodyDelay62/1 -> b(62)/1, BodyDelay63/1
  b(62)/1 -> BodyLSum62/1
  BodyLSum62/1 -> BodyLSum63/2
  BodyDelay63/1 -> b(63)/1, BodyDelay64/1
  b(63)/1 -> BodyLSum63/1
  BodyLSum63/1 -> BodyLSum64/2
  BodyDelay64/1 -> b(64)/1, BodyDelay65/1
  b(64)/1 -> BodyLSum64/1
  BodyLSum64/1 -> BodyLSum65/2
  BodyDelay65/1 -> b(65)/1, BodyDelay66/1
  b(65)/1 -> BodyLSum65/1
  BodyLSum65/1 -> BodyLSum66/2
  BodyDelay66/1 -> b(66)/1, BodyDelay67/1
  b(66)/1 -> BodyLSum66/1
  BodyLSum66/1 -> BodyLSum67/2
  BodyDelay67/1 -> b(67)/1, BodyDelay68/1
  b(67)/1 -> BodyLSum67/1
  BodyLSum67/1 -> BodyLSum68/2
  BodyDelay68/1 -> b(68)/1, BodyDelay69/1
  b(68)/1 -> BodyLSum68/1
  BodyLSum68/1 -> BodyLSum69/2
  BodyDelay69/1 -> b(69)/1, BodyDelay70/1
  b(69)/1 -> BodyLSum69/1
  BodyLSum69/1 -> BodyLSum70/2
  BodyDelay70/1 -> b(70)/1, BodyDelay71/1
  b(70)/1 -> BodyLSum70/1
  BodyLSum70/1 -> BodyLSum71/2
  BodyDelay71/1 -> b(71)/1, BodyDelay72/1
  b(71)/1 -> BodyLSum71/1
  BodyLSum71/1 -> BodyLSum72/2
  BodyDelay72/1 -> b(72)/1, BodyDelay73/1
  b(72)/1 -> BodyLSum72/1
  BodyLSum72/1 -> BodyLSum73/2
  BodyDelay73/1 -> b(73)/1, BodyDelay74/1
  b(73)/1 -> BodyLSum73/1
  BodyLSum73/1 -> BodyLSum74/2
  BodyDelay74/1 -> b(74)/1, BodyDelay75/1
  b(74)/1 -> BodyLSum74/1
  BodyLSum74/1 -> BodyLSum75/2
  BodyDelay75/1 -> b(75)/1, BodyDelay76/1
  b(75)/1 -> BodyLSum75/1
  BodyLSum75/1 -> BodyLSum76/2
  BodyDelay76/1 -> b(76)/1, BodyDelay77/1
  b(76)/1 -> BodyLSum76/1
  BodyLSum76/1 -> BodyLSum77/2
  BodyDelay77/1 -> b(77)/1, BodyDelay78/1
  b(77)/1 -> BodyLSum77/1
  BodyLSum77/1 -> BodyLSum78/2
  BodyDelay78/1 -> b(78)/1, BodyDelay79/1
  b(78)/1 -> BodyLSum78/1
  BodyLSum78/1 -> BodyLSum79/2
  BodyDelay79/1 -> b(79)/1, BodyDelay80/1
  b(79)/1 -> BodyLSum79/1
  BodyLSum79/1 -> BodyLSum80/2
  BodyDelay80/1 -> b(80)/1, BodyDelay81/1
  b(80)/1 -> BodyLSum80/1
  BodyLSum80/1 -> BodyLSum81/2
  BodyDelay81/1 -> b(81)/1, BodyDelay82/1
  b(81)/1 -> BodyLSum81/1
  BodyLSum81/1 -> BodyLSum82/2
  BodyDelay82/1 -> b(82)/1, BodyDelay83/1
  b(82)/1 -> BodyLSum82/1
  BodyLSum82/1 -> BodyLSum83/2
  BodyDelay83/1 -> b(83)/1, BodyDelay84/1
  b(83)/1 -> BodyLSum83/1
  BodyLSum83/1 -> BodyLSum84/2
  BodyDelay84/1 -> b(84)/1, BodyDelay85/1
  b(84)/1 -> BodyLSum84/1
  BodyLSum84/1 -> BodyLSum85/2
  BodyDelay85/1 -> b(85)/1, BodyDelay86/1
  b(85)/1 -> BodyLSum85/1
  BodyLSum85/1 -> BodyLSum86/2
  BodyDelay86/1 -> b(86)/1, BodyDelay87/1
  b(86)/1 -> BodyLSum86/1
  BodyLSum86/1 -> BodyLSum87/2
  BodyDelay87/1 -> b(87)/1, BodyDelay88/1
  b(87)/1 -> BodyLSum87/1
  BodyLSum87/1 -> BodyLSum88/2
  BodyDelay88/1 -> b(88)/1, BodyDelay89/1
  b(88)/1 -> BodyLSum88/1
  BodyLSum88/1 -> BodyLSum89/2
  BodyDelay89/1 -> b(89)/1, BodyDelay90/1
  b(89)/1 -> BodyLSum89/1
  BodyLSum89/1 -> BodyLSum90/2
  BodyDelay90/1 -> b(90)/1, BodyDelay91/1
  b(90)/1 -> BodyLSum90/1
  BodyLSum90/1 -> BodyLSum91/2
  BodyDelay91/1 -> b(91)/1, BodyDelay92/1
  b(91)/1 -> BodyLSum91/1
  BodyLSum91/1 -> BodyLSum92/2
  BodyDelay92/1 -> b(92)/1, BodyDelay93/1
  b(92)/1 -> BodyLSum92/1
  BodyLSum92/1 -> BodyLSum93/2
  BodyDelay93/1 -> b(93)/1, BodyDelay94/1
  b(93)/1 -> BodyLSum93/1
  BodyLSum93/1 -> BodyLSum94/2
  BodyDelay94/1 -> b(94)/1, BodyDelay95/1
  b(94)/1 -> BodyLSum94/1
  BodyLSum94/1 -> BodyLSum95/2
  BodyDelay95/1 -> b(95)/1, BodyDelay96/1
  b(95)/1 -> BodyLSum95/1
  BodyLSum95/1 -> BodyLSum96/2
  BodyDelay96/1 -> b(96)/1, BodyDelay97/1
  b(96)/1 -> BodyLSum96/1
  BodyLSum96/1 -> BodyLSum97/2
  BodyDelay97/1 -> b(97)/1, BodyDelay98/1
  b(97)/1 -> BodyLSum97/1
  BodyLSum97/1 -> BodyLSum98/2
  BodyDelay98/1 -> b(98)/1, BodyDelay99/1
  b(98)/1 -> BodyLSum98/1
  BodyLSum98/1 -> BodyLSum99/2
  BodyDelay99/1 -> b(99)/1, BodyDelay100/1
  b(99)/1 -> BodyLSum99/1
  BodyLSum99/1 -> BodyLSum100/2
  BodyDelay100/1 -> b(100)/1, BodyDelay101/1
  b(100)/1 -> BodyLSum100/1
  BodyLSum100/1 -> BodyLSum101/1
  BodyDelay101/1 -> b(101)/1
  b(101)/1 -> BodyLSum101/2
  BodyLSum101/1 -> Output/1
